simulink model "Projekat_pod_b_simulink"  (R2024b)
settings: Solver=ode23tb  StartTime=0.0  StopTime=10.0  RelTol=1e-3
settings Model: Creator=HP  LastModifiedBy=HP

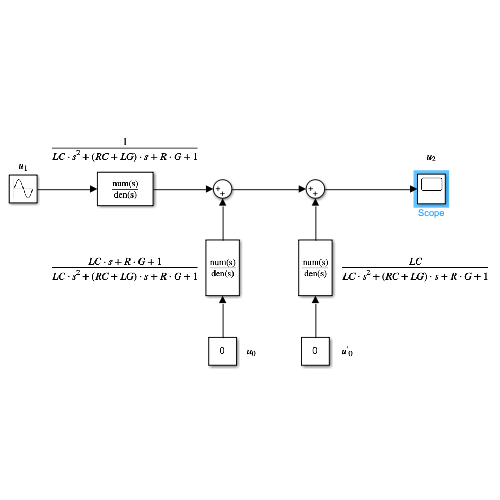
[thumbnail: Simulink's stored preview of the top-level diagram]
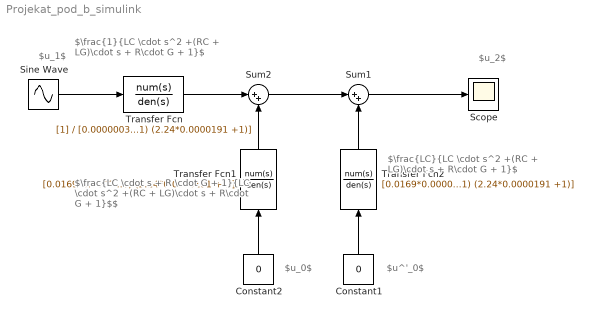
== system Projekat_pod_b_simulink ==
  note: $\frac{LC \cdot s + R \cdot G + 1}{LC \cdot s^2 +(RC + LG)\cdot s + R\cdot G + 1}$$
  note: $\frac{1}{LC \cdot s^2 +(RC + LG)\cdot s + R\cdot G + 1}$
  note: $u_2$
  note: $u^'_0$
  note: $u_0$
  note: $u_1$
  note: $\frac{LC}{LC \cdot s^2 +(RC + LG)\cdot s + R\cdot G + 1}$
  Constant1 : Constant  Value=0
  Constant2 : Constant  Value=0
  Scope : Scope
  Sine Wave : Sin  Amplitude=35000 * sqrt(2)  Frequency=2*pi*50  Phase=pi/2  SampleTime=0
  Sum1 : Sum  Inputs=|++
  Sum2 : Sum  Inputs=|++
  Transfer Fcn : TransferFcn  Denominator=[0.000000382*0.0169 (2.24*0.000000382 + 0.0169*0.0000191) (2.24*0.0000191 +1)]
  Transfer Fcn1 : TransferFcn  Numerator=[0.0169*0.000000382 (2.24*0.0000191 +1)]  Denominator=[0.000000382*0.0169 (2.24*0.000000382 + 0.0169*0.0000191) (2.24*0.0000191 +1)]
  Transfer Fcn2 : TransferFcn  Numerator=[0.0169*0.000000382]  Denominator=[0.000000382*0.0169 (2.24*0.000000382 + 0.0169*0.0000191) (2.24*0.0000191 +1)]
  wires:
  Sine Wave/1 -> Transfer Fcn/1
  Constant2/1 -> Transfer Fcn1/1
  Transfer Fcn/1 -> Sum2/1
  Transfer Fcn1/1 -> Sum2/2
  Sum2/1 -> Sum1/1
  Constant1/1 -> Transfer Fcn2/1
  Transfer Fcn2/1 -> Sum1/2
  Sum1/1 -> Scope/1
